simulink model "PM_fnc12_TestHarness"  (R2022a)
settings: Solver=FixedStepDiscrete  StartTime=1  StopTime=inf  FixedStep=1  RelTol=1e-3
values from neighbouring files (symbols this model uses):
  fixedsteprate_s = rate_s    (= 0.01)    [PM_fnc1000_tc01_iter01_testsignal_builder.m]    (also in PM_fnc21_tc01_iter01_testsignal_builder.m; PM_fnc22_tc01_iter01_testsignal_builder.m)
undefined symbols (not defined in the file or in its folder): cal_DchgPL1_expiry_dur_thresh_ms, cal_DchgPL1_restore_dur_thresh_ms, cal_DchgPL2_amps_thresh_mA, cal_DchgPL2_expiry_dur_thresh_ms, cal_DchgPL2_restore_dur_thresh_ms
settings Model: PacingRate=3  Creator=306427  LastModifiedBy=306427
settings SolverCC: ZeroCrossAlgorithm=Adaptive

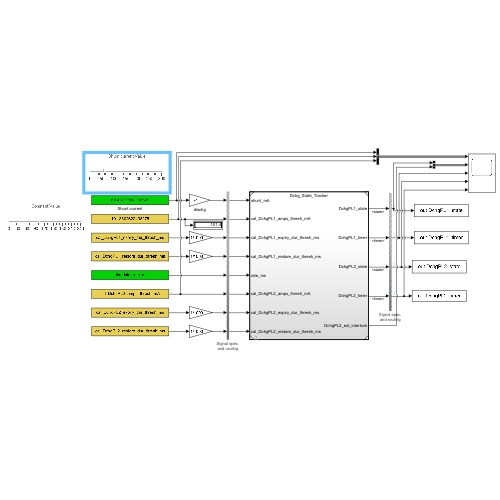
[thumbnail: Simulink's stored preview of the top-level diagram]
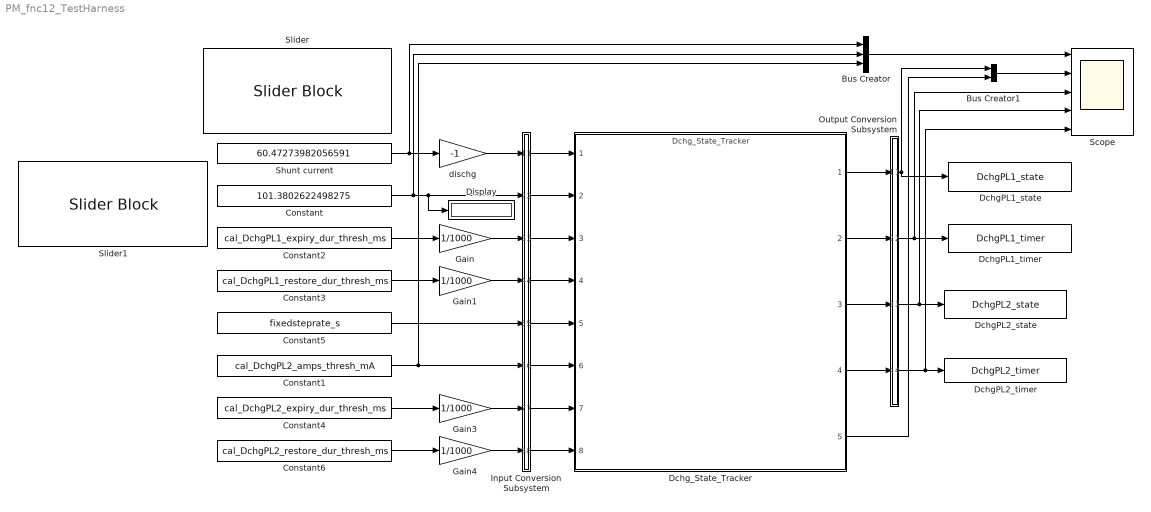
== system PM_fnc12_TestHarness ==
  Bus Creator : BusCreator  Inputs=3
  Bus Creator1 : BusCreator  Inputs=2
  Constant : Constant  Value=101.3802622498275
  Constant1 : Constant  Value=cal_DchgPL2_amps_thresh_mA
  Constant2 : Constant  Value=cal_DchgPL1_expiry_dur_thresh_ms
  Constant3 : Constant  Value=cal_DchgPL1_restore_dur_thresh_ms
  Constant4 : Constant  Value=cal_DchgPL2_expiry_dur_thresh_ms
  Constant5 : Constant  Value=fixedsteprate_s
  Constant6 : Constant  Value=cal_DchgPL2_restore_dur_thresh_ms
  DchgPL1_state : ToWorkspace  VariableName=DchgPL1_state
      settings: Save2DSignal=2-D array (concatenate along first dimension)
  DchgPL1_timer : ToWorkspace  VariableName=DchgPL1_timer
      settings: Save2DSignal=2-D array (concatenate along first dimension)
  DchgPL2_state : ToWorkspace  VariableName=DchgPL2_state
      settings: Save2DSignal=2-D array (concatenate along first dimension)
  DchgPL2_timer : ToWorkspace  VariableName=DchgPL2_timer
      settings: Save2DSignal=2-D array (concatenate along first dimension)
  Dchg_State_Tracker : ModelReference  ModelNameDialog=Dchg_State_Tracker  SimulationMode=Normal  ModelReferenceVersion=1.14
  Display : Display
  Gain{,1,3..4} (4 alike) : Gain  Gain=1/1000
  Input Conversion Subsystem : Subsystem  Tag=__SLT_ICS__  Description=|
      | Signal spec.
      | and routing
      settings: AttributesFormatString=%<Description>
  Output Conversion Subsystem : Subsystem  Tag=__SLT_OCS__  Description=|
      | Signal spec.
      | and routing
      settings: AttributesFormatString=%<Description>
  Scope : Scope  NumInputPorts=5
  Shunt current : Constant  Value=60.47273982056591
  Slider : SliderBlock  ScaleMax=300
  Slider1 : SliderBlock  ScaleMax=240
  dischg : Gain  Gain=-1
  wires:
  Shunt current/1 -> dischg/1, Bus Creator/1
  Constant/1 -> Display/1, Input Conversion Subsystem/2(Inport_2), Bus Creator/2
  Constant2/1 -> Gain/1
  Constant3/1 -> Gain1/1
  Constant5/1 -> Input Conversion Subsystem/5(Inport_5)
  Constant4/1 -> Gain3/1
  Constant6/1 -> Gain4/1
  Output Conversion Subsystem/1(Outport_1) -> Bus Creator1/1, DchgPL1_state/1
  Output Conversion Subsystem/2(Outport_2) -> DchgPL1_timer/1, Scope/3
  Output Conversion Subsystem/3(Outport_3) -> DchgPL2_state/1, Scope/4
  Output Conversion Subsystem/4(Outport_4) -> DchgPL2_timer/1, Scope/5
  Input Conversion Subsystem/1(Outport_1) -> Dchg_State_Tracker/1
  Input Conversion Subsystem/2(Outport_2) -> Dchg_State_Tracker/2
  Input Conversion Subsystem/3(Outport_3) -> Dchg_State_Tracker/3
  Input Conversion Subsystem/4(Outport_4) -> Dchg_State_Tracker/4
  Input Conversion Subsystem/5(Outport_5) -> Dchg_State_Tracker/5
  Input Conversion Subsystem/6(Outport_6) -> Dchg_State_Tracker/6
  Input Conversion Subsystem/7(Outport_7) -> Dchg_State_Tracker/7
  Input Conversion Subsystem/8(Outport_8) -> Dchg_State_Tracker/8
  Dchg_State_Tracker/1 -> Output Conversion Subsystem/1(Inport_1)
  Dchg_State_Tracker/2 -> Output Conversion Subsystem/2(Inport_2)
  Dchg_State_Tracker/3 -> Output Conversion Subsystem/3(Inport_3)
  Dchg_State_Tracker/4 -> Output Conversion Subsystem/4(Inport_4)
  Gain/1 -> Input Conversion Subsystem/3(Inport_3)
  Gain1/1 -> Input Conversion Subsystem/4(Inport_4)
  Constant1/1 -> Input Conversion Subsystem/6(Inport_6), Bus Creator/3
  Gain3/1 -> Input Conversion Subsystem/7(Inport_7)
  Gain4/1 -> Input Conversion Subsystem/8(Inport_8)
  dischg/1 -> Input Conversion Subsystem/1(Inport_1)
  Bus Creator/1 -> Scope/1
  Bus Creator1/1 -> Scope/2
  Dchg_State_Tracker/5 -> Bus Creator1/2

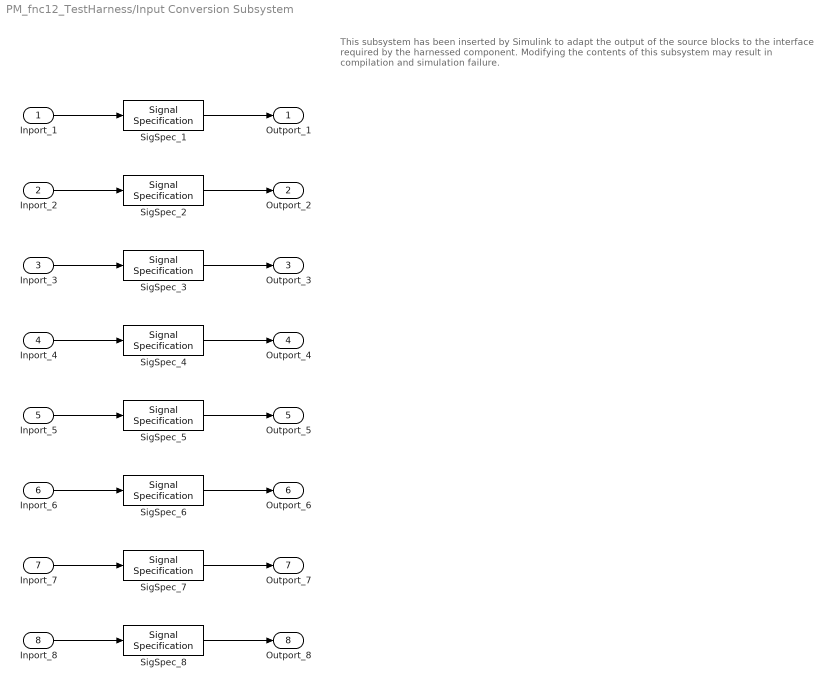
== system PM_fnc12_TestHarness/Input Conversion Subsystem ==
  note: This subsystem has been inserted by Simulink to adapt the output of the source blocks to the interface required by the harnessed component.
      |  Modifying the contents of this subsystem may result in compilation and simulation failure.
  Inport_1 : Inport
  Inport_2 : Inport  Port=2
  Inport_3 : Inport  Port=3
  Inport_4 : Inport  Port=4
  Inport_5 : Inport  Port=5
  Inport_6 : Inport  Port=6
  Inport_7 : Inport  Port=7
  Inport_8 : Inport  Port=8
  SigSpec_{1..8} (8 alike) : SignalSpecification  OutDataTypeStr=double  Dimensions=[1]  SampleTime=[-1, 0]
  Outport_1 : Outport
  Outport_2 : Outport  Port=2
  Outport_3 : Outport  Port=3
  Outport_4 : Outport  Port=4
  Outport_5 : Outport  Port=5
  Outport_6 : Outport  Port=6
  Outport_7 : Outport  Port=7
  Outport_8 : Outport  Port=8
  wires:
  SigSpec_1/1 -> Outport_1/1
  Inport_1/1 -> SigSpec_1/1
  SigSpec_2/1 -> Outport_2/1
  Inport_2/1 -> SigSpec_2/1
  SigSpec_3/1 -> Outport_3/1
  Inport_3/1 -> SigSpec_3/1
  SigSpec_4/1 -> Outport_4/1
  Inport_4/1 -> SigSpec_4/1
  SigSpec_5/1 -> Outport_5/1
  Inport_5/1 -> SigSpec_5/1
  SigSpec_6/1 -> Outport_6/1
  Inport_6/1 -> SigSpec_6/1
  SigSpec_7/1 -> Outport_7/1
  Inport_7/1 -> SigSpec_7/1
  SigSpec_8/1 -> Outport_8/1
  Inport_8/1 -> SigSpec_8/1

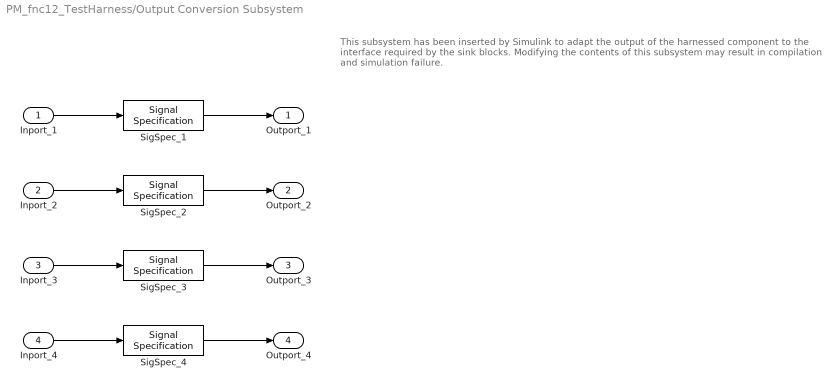
== system PM_fnc12_TestHarness/Output Conversion Subsystem ==
  note: This subsystem has been inserted by Simulink to adapt the output of the harnessed component to the interface required by the sink blocks.
      |  Modifying the contents of this subsystem may result in compilation and simulation failure.
  Inport_1 : Inport
  Inport_2 : Inport  Port=2
  Inport_3 : Inport  Port=3
  Inport_4 : Inport  Port=4
  SigSpec_{1..4} (4 alike) : SignalSpecification  OutDataTypeStr=double  Dimensions=[1]
  Outport_1 : Outport
  Outport_2 : Outport  Port=2
  Outport_3 : Outport  Port=3
  Outport_4 : Outport  Port=4
  wires:
  Inport_1/1 -> SigSpec_1/1
  SigSpec_1/1 -> Outport_1/1
  Inport_2/1 -> SigSpec_2/1
  SigSpec_2/1 -> Outport_2/1
  Inport_3/1 -> SigSpec_3/1
  SigSpec_3/1 -> Outport_3/1
  Inport_4/1 -> SigSpec_4/1
  SigSpec_4/1 -> Outport_4/1
